simulink model "ReactionWheels_Model"  (R2023a)
settings: Solver=VariableStepAuto  StartTime=0.0  StopTime=50  RelTol=1e-3
values from neighbouring files (symbols this model uses):
  A_motor = [-B/J Kt/J ... (first row only)    [State_Space_RW.m]
  B = (1/438)*(60/(2*pi))*1e-3    (= 2.18020469989e-05)    [State_Space_RW.m]
  B_motor = [0; 1/La]    [State_Space_RW.m]
  C_motor = [0 Kt]    [State_Space_RW.m]
  D_motor = 0    [State_Space_RW.m]
  J = J_rotor+ J_flywheel    (= 7.1569e-05)    [State_Space_RW.m]
  Ke = (1/1120)*(60/(2*pi))    (= 0.00852615766564)    [State_Space_RW.m]
  Kt = 8.55e-3    (= 0.00855)    [State_Space_RW.m]
  La = 0.222e-3    (= 0.000222)    [State_Space_RW.m]
  Ra = 3.36    [State_Space_RW.m]
settings Model: Creator=Personal  LastModifiedBy=Personal

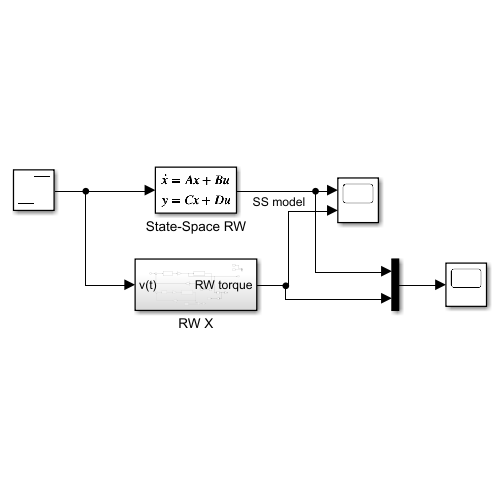
[thumbnail: Simulink's stored preview of the top-level diagram]
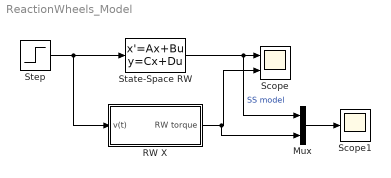
== system ReactionWheels_Model ==
  Mux : Mux  Inputs=2
  RW X : Subsystem
  Scope : Scope  NumInputPorts=2
  Scope1 : Scope
  State-Space RW : StateSpace  A=A_motor  B=B_motor  C=C_motor  D=D_motor  InitialCondition=0
  Step : Step  Time=3  After=6  SampleTime=0
  wires:
  Step/1 -> RW X/1(v(t)), State-Space RW/1
  State-Space RW/1 -> Mux/1, Scope/1  "SS model"
  RW X/1(RW torque) -> Mux/2, Scope/2
  Mux/1 -> Scope1/1

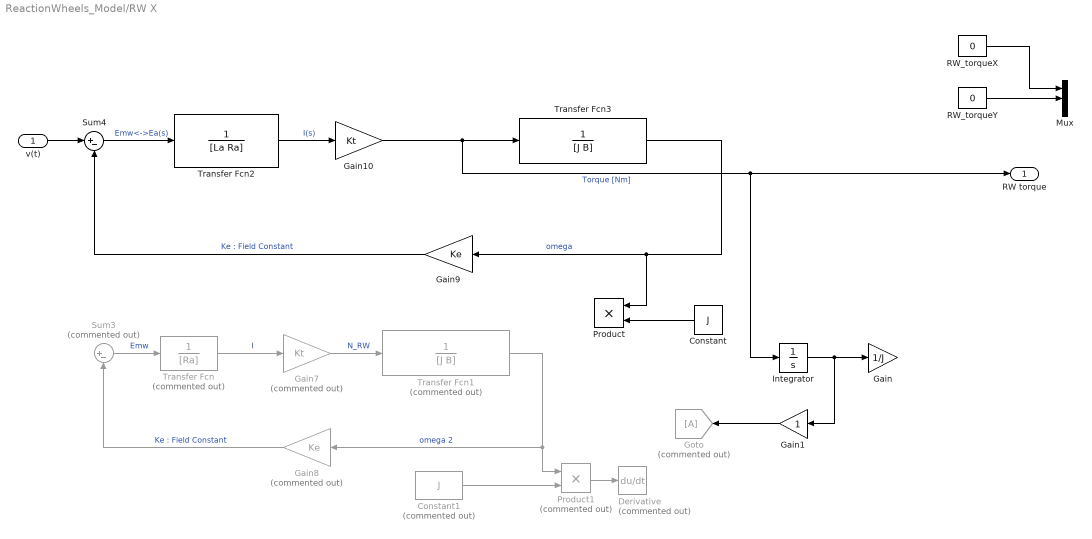
== system ReactionWheels_Model/RW X ==
  v(t) : Inport
  Constant : Constant  Value=J
  Constant1 : Constant  Commented=on  Value=J
  Derivative : Derivative  Commented=on
  Gain : Gain  Gain=1/J
  Gain1 : Gain
  Gain10 : Gain  Gain=Kt
  Gain7 : Gain  Commented=on  Gain=Kt
  Gain8 : Gain  Commented=on  Gain=Ke
  Gain9 : Gain  Gain=Ke
  Goto : Goto  Commented=on
  Integrator : Integrator
  Mux : Mux  Inputs=3
  Product : Product
  Product1 : Product  Commented=on
  RW_torqueX : Constant  Value=0
  RW_torqueY : Constant  Value=0
  Sum3 : Sum  Commented=on  Inputs=|+-
  Sum4 : Sum  Inputs=|+-
  Transfer Fcn : TransferFcn  Commented=on  Denominator=[Ra]
  Transfer Fcn1 : TransferFcn  Commented=on  Denominator=[J B]
  Transfer Fcn2 : TransferFcn  Denominator=[La Ra]
  Transfer Fcn3 : TransferFcn  Denominator=[J B]
  RW torque : Outport  VectorParamsAs1DForOutWhenUnconnected=off
  wires:
  Gain1/1 -> Goto/1
  Gain10/1 -> Transfer Fcn3/1, Integrator/1, RW torque/1  "Torque [Nm]"
  RW_torqueY/1 -> Mux/2
  RW_torqueX/1 -> Mux/1
  Gain8/1 -> Sum3/2  "Ke : Field Constant"
  Transfer Fcn/1 -> Gain7/1  "I"
  Sum3/1 -> Transfer Fcn/1  "Emw"
  Gain7/1 -> Transfer Fcn1/1  "N_RW"
  Transfer Fcn1/1 -> Gain8/1, Product1/1  "omega 2"
  Constant1/1 -> Product1/2
  Product1/1 -> Derivative/1
  v(t)/1 -> Sum4/1
  Integrator/1 -> Gain/1, Gain1/1
  Constant/1 -> Product/2
  Transfer Fcn3/1 -> Product/1, Gain9/1  "omega"
  Gain9/1 -> Sum4/2  "Ke : Field Constant"
  Sum4/1 -> Transfer Fcn2/1  "Emw<->Ea(s)"
  Transfer Fcn2/1 -> Gain10/1  "I(s)"
